simulink model "test_PCI6052E_20130416_3ch"  (Simulink 7.7)
settings: Solver=ode4  StartTime=0.0  StopTime=inf  RelTol=1e-3
PreLoadFcn:
  | % Here are parameters fixed
  | % during running the real-time programs.
  | %
  | winLen=256;
  | ana_hopSize=44;
  | syn_hopSize=90;
  | 
  | nFFT=1024;
  | SampRate=44100;
  | Ts=1/SampRate;
  | 
  | % % now encoded in RealSong_control
  | %cepst_nfft=2048;    % nfft size for cepstrum.
  | %
  | %up_pitch= 8000;%
  | %low_pitch=400;%
  | %
  | %quefrency = [0:cepst_nfft]'*nFFT/(SampRate*cepst_nfft); % quefrency in [sec].
  | %quefrency_index=find((1./quefrency<up_pitch & 1./quefrency > low_pitch)); % select quefrency in 400 to 8000 Hz range.
  | 
  | 
  | %frange=[400,8000];
  | %f=SampRate*((1:nFFT)-1)/nFFT;
  | %findex=find(f>=frange(1)&f<=frange(2));
  | %entropy_frange=[1000,8000];
  | %efindex=find(f>=entropy_frange(1)&f<=entropy_frange(2));
  | 
  | 
  | mingap=1;
  | minsyl =6;
values from neighbouring files (symbols this model uses):
  amp_thresh = str2double(get(handles.edit_amp_thresh,'String'))    [RealSong_control_013.m]
  efindex = find(f>=efrange(1)&f<=efrange(2))    [RealSong_control_013.m]
  findex = find(f>=pm.frange(1)&f<=pm.frange(2))    [RealSong_control_013.m]
  mainsyl = varargin{1}    [RealSong_control_013.m]
  quefrency_index = find((1./quefrency<up_pitch & 1./quefrency > low_pitch))    [RealSong_control_013.m]
  scaling_factor = presyl.template_scaling_factor    [RealSong_control_013.m]
undefined symbols (not defined in the file or in its folder): AO1_TTL_Freq, dfilt, init_stim_vector, maindetection_startcnt, maintarget_spectrum_filter, max_presyl_cancel_counter, presyl_cntmin, svmdata
libraries: simulink x13, dspsigops x4, xpcnilib x3, dsparch4 x2, dspxfrm3 x2
(part 2 of 2)

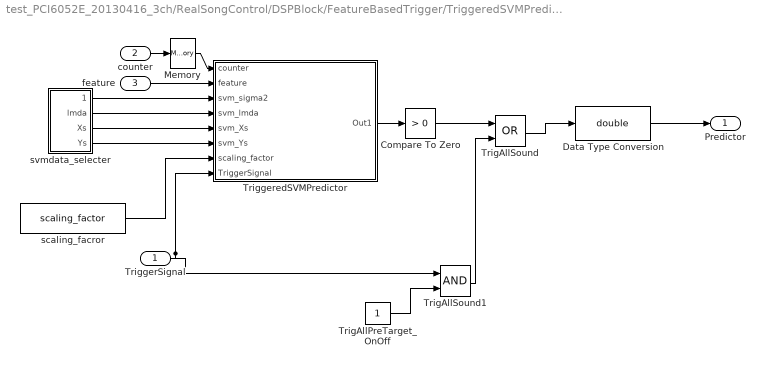
== system test_PCI6052E_20130416_3ch/RealSongControl/DSPBlock/FeatureBasedTrigger/TriggeredSVMPredictor ==
  TriggerSignal : Inport
  counter : Inport  Port=2
  feature : Inport  Port=3
  Compare To Zero : simulink/Logic and Bit Operations/Compare To Zero  SystemSampleTime=-1  relop=>  LogicOutDataTypeMode=uint8
  Data Type Conversion : DataTypeConversion  OutDataTypeStr=double
  Memory : Memory  InheritSampleTime=on
  TrigAllPreTarget_OnOff : Constant  VectorParams1D=off
  TrigAllSound : Logic  Operator=OR  AllPortsSameDT=off  OutDataTypeStr=boolean
  TrigAllSound1 : Logic  AllPortsSameDT=off  OutDataTypeStr=boolean
  TriggeredSVMPredictor : Subsystem  TreatAsAtomicUnit=on
  scaling_facror : Constant  Value=scaling_factor
  svmdata_selecter : Subsystem  mask{svmdata=svmdata}
      mask prompts: svmdata "svm data"
  Predictor : Outport
  wires:
  scaling_facror/1 -> TriggeredSVMPredictor/7(scaling_factor)
  svmdata_selecter/1(sigma2) -> TriggeredSVMPredictor/3(svm_sigma2)
  svmdata_selecter/2(lmda) -> TriggeredSVMPredictor/4(svm_lmda)
  svmdata_selecter/3(Xs) -> TriggeredSVMPredictor/5(svm_Xs)
  svmdata_selecter/4(Ys) -> TriggeredSVMPredictor/6(svm_Ys)
  counter/1 -> Memory/1
  feature/1 -> TriggeredSVMPredictor/2(feature)
  TriggeredSVMPredictor/1(Out1) -> Compare To Zero/1
  TriggerSignal/1 -> TriggeredSVMPredictor/8(TriggerSignal), TrigAllSound1/1
  Memory/1 -> TriggeredSVMPredictor/1(counter)
  Data Type Conversion/1 -> Predictor/1
  Compare To Zero/1 -> TrigAllSound/1
  TrigAllSound/1 -> Data Type Conversion/1
  TrigAllPreTarget_OnOff/1 -> TrigAllSound1/2
  TrigAllSound1/1 -> TrigAllSound/2

== system test_PCI6052E_20130416_3ch/RealSongControl/DSPBlock/FeatureBasedTrigger/amplitude triggered  Iterative_mean_var ==
  note: 1: entropy
      | 2: FM
      | 3: frequency
      | 4: pitch
      | 5: pitchgoodness
  amp : Inport
  features : Inport  Port=2
  amp_thresh : Inport  Port=3
  AboveAmplitudeDetectionAndCounter1 : Subsystem  mask{mingap=mingap, minsyl=minsyl}
      mask prompts: mingap "Gap shorter than this is neglected"; minsyl "On state must be longer than this"
  AboveSyllableCounter : Subsystem
  Iterative_mean_var : Stateflow chart  TreatAsAtomicUnit=on
  on_signal : Outport
  syl_duration : Outport  Port=2
  meanvar : Outport  Port=3
  wires:
  Iterative_mean_var/1(out) -> meanvar/1
  features/1 -> Iterative_mean_var/1(x)
  amp/1 -> AboveAmplitudeDetectionAndCounter1/1(Input)
  amp_thresh/1 -> AboveAmplitudeDetectionAndCounter1/2(threshold)
  AboveAmplitudeDetectionAndCounter1/1(SignalOn) -> Iterative_mean_var/2(on_signal), on_signal/1, AboveSyllableCounter/1(LogicalInput)
  AboveSyllableCounter/1(count) -> syl_duration/1

== system test_PCI6052E_20130416_3ch/RealSongControl/DSPBlock/SoundOnOffCounter/SoundOffCounter ==
  LogicalInput : Inport
  Counter : Subsystem  TreatAsAtomicUnit=on
  Data Type Conversion1 : DataTypeConversion  OutDataTypeStr=double  RndMeth=Zero
  count : Outport
  wires:
  Data Type Conversion1/1 -> Counter/1(In1)
  LogicalInput/1 -> Data Type Conversion1/1, Counter/Enable
  Counter/1(Out1) -> count/1

== system test_PCI6052E_20130416_3ch/RealSongControl/DSPBlock/SoundOnOffCounter/SoundOnCounter ==
  LogicalInput : Inport
  Counter : Subsystem  TreatAsAtomicUnit=on
  Data Type Conversion1 : DataTypeConversion  OutDataTypeStr=double  RndMeth=Zero
  count : Outport
  wires:
  Data Type Conversion1/1 -> Counter/1(In1)
  LogicalInput/1 -> Data Type Conversion1/1, Counter/Enable
  Counter/1(Out1) -> count/1

== system test_PCI6052E_20130416_3ch/RealSongControl/DSPBlock/BoutCounter/BoutDurCounter/CorrectDelayedPulseGenerator ForSyllableOn ==
  trig : Inport
  DSP Constant2 : Constant  Value=maindetection_startcnt  VectorParams1D=off
  DSP Constant3 : Constant  Value=width  VectorParams1D=off
  Delayed TTL generator : Stateflow chart  TreatAsAtomicUnit=on
  TTL : Outport
  wires:
  DSP Constant2/1 -> Delayed TTL generator/2(delays)
  DSP Constant3/1 -> Delayed TTL generator/3(width)
  trig/1 -> Delayed TTL generator/1(trig)
  Delayed TTL generator/1(out) -> TTL/1

== system test_PCI6052E_20130416_3ch/RealSongControl/DSPBlock/BoutCounter/BoutDurCounter/PreSoundOnCounter ==
  LogicalInput : Inport
  Counter : Subsystem  TreatAsAtomicUnit=on
  Data Type Conversion1 : DataTypeConversion  OutDataTypeStr=double  RndMeth=Zero
  count : Outport
  wires:
  Data Type Conversion1/1 -> Counter/1(In1)
  LogicalInput/1 -> Data Type Conversion1/1, Counter/Enable
  Counter/1(Out1) -> count/1

== system test_PCI6052E_20130416_3ch/RealSongControl/DSPBlock/BoutCounter/BoutDurCounter/SoundOnCounter ==
  LogicalInput : Inport
  Counter : Subsystem  TreatAsAtomicUnit=on
  Data Type Conversion1 : DataTypeConversion  OutDataTypeStr=double  RndMeth=Zero
  count : Outport
  wires:
  Data Type Conversion1/1 -> Counter/1(In1)
  LogicalInput/1 -> Data Type Conversion1/1, Counter/Enable
  Counter/1(Out1) -> count/1

== system test_PCI6052E_20130416_3ch/RealSongControl/DSPBlock/FeatureBasedTrigger/MainDetectCounter/Counter ==
  In1 : Inport
  Enable : EnablePort  StatesWhenEnabling=reset
  Memory1 : Memory  InheritSampleTime=on
  Sum1 : Sum  Inputs=|++  SaturateOnIntegerOverflow=on
  Out1 : Outport  OutputWhenDisabled=reset  InitialOutput=0
  wires:
  In1/1 -> Sum1/1
  Sum1/1 -> Out1/1, Memory1/1
  Memory1/1 -> Sum1/2

== system test_PCI6052E_20130416_3ch/RealSongControl/DSPBlock/FeatureBasedTrigger/PreSyllableDetectionAtEndOfSyllable/CancelCounter ==
  LogicalInput : Inport
  Counter : Subsystem  TreatAsAtomicUnit=on
  Data Type Conversion1 : DataTypeConversion  OutDataTypeStr=double  RndMeth=Zero
  count : Outport
  wires:
  Data Type Conversion1/1 -> Counter/1(In1)
  LogicalInput/1 -> Data Type Conversion1/1, Counter/Enable
  Counter/1(Out1) -> count/1

== system test_PCI6052E_20130416_3ch/RealSongControl/DSPBlock/FeatureBasedTrigger/PreSyllableDetectionAtEndOfSyllable/EnabledKeepMaxCounter ==
  enable : Inport
  binarysignal : Inport  Port=2
  EnabledMaxCounter : Subsystem  TreatAsAtomicUnit=on
  SyllableCounter : Subsystem
  MaxCount : Outport
  wires:
  SyllableCounter/1(count) -> EnabledMaxCounter/1(In1)
  enable/1 -> EnabledMaxCounter/Enable
  EnabledMaxCounter/1(Out1) -> MaxCount/1
  binarysignal/1 -> SyllableCounter/1(LogicalInput)

== system test_PCI6052E_20130416_3ch/RealSongControl/DSPBlock/FeatureBasedTrigger/RndCatchMainGateWindow/CorrectDelayedPulseGenerator ==
  trig : Inport
  delay : Inport  Port=2
  width : Inport  Port=3
  Delayed TTL generator : Stateflow chart  TreatAsAtomicUnit=on
  TTL : Outport
  wires:
  delay/1 -> Delayed TTL generator/2(delays)
  width/1 -> Delayed TTL generator/3(width)
  trig/1 -> Delayed TTL generator/1(trig)
  Delayed TTL generator/1(out) -> TTL/1

== system test_PCI6052E_20130416_3ch/RealSongControl/DSPBlock/FeatureBasedTrigger/RndCatchMainGateWindow/CorrectDelayedPulseGenerator1 ==
  trig : Inport
  delay : Inport  Port=2
  width : Inport  Port=3
  Delayed TTL generator : Stateflow chart  TreatAsAtomicUnit=on
  TTL : Outport
  wires:
  delay/1 -> Delayed TTL generator/2(delays)
  width/1 -> Delayed TTL generator/3(width)
  trig/1 -> Delayed TTL generator/1(trig)
  Delayed TTL generator/1(out) -> TTL/1

== system test_PCI6052E_20130416_3ch/RealSongControl/DSPBlock/FeatureBasedTrigger/RndCatchMainGateWindow/EnabledCatchSignalBox ==
  In1 : Inport
  Enable : EnablePort
  CatchLine : Logic  Operator=NOT  AllPortsSameDT=off  OutDataTypeStr=boolean
  CatchRatioConstant : Constant  Value=0
  PreSyllableDetection : Logic  AllPortsSameDT=off  OutDataTypeStr=boolean
  Relational Operator : RelationalOperator  Operator=<=  OutDataTypeStr=boolean
  Uniform Random Number : UniformRandomNumber  Minimum=0
  Hit : Outport  OutputWhenDisabled=reset  InitialOutput=0
  Catch : Outport  Port=2  OutputWhenDisabled=reset  InitialOutput=0
  wires:
  CatchRatioConstant/1 -> Relational Operator/1
  Uniform Random Number/1 -> Relational Operator/2
  PreSyllableDetection/1 -> Hit/1, CatchLine/1
  In1/1 -> PreSyllableDetection/1
  Relational Operator/1 -> PreSyllableDetection/2
  CatchLine/1 -> Catch/1

== system test_PCI6052E_20130416_3ch/RealSongControl/DSPBlock/FeatureBasedTrigger/TriggeredSVMPredictor/TriggeredSVMPredictor ==
  counter : Inport
  feature : Inport  Port=2
  svm_sigma2 : Inport  Port=3
  svm_lmda : Inport  Port=4
  svm_Xs : Inport  Port=5
  svm_Ys : Inport  Port=6
  scaling_factor : Inport  Port=7
  TriggerSignal : Inport  Port=8
  svm_predict : Stateflow chart  TreatAsAtomicUnit=on
  Out1 : Outport
  wires:
  counter/1 -> svm_predict/1(counter)
  svm_predict/1(predictor) -> Out1/1
  feature/1 -> svm_predict/2(feature)
  svm_sigma2/1 -> svm_predict/3(svm_sigma2)
  svm_lmda/1 -> svm_predict/4(svm_lmda)
  svm_Xs/1 -> svm_predict/5(svm_Xs)
  svm_Ys/1 -> svm_predict/6(svm_Ys)
  scaling_factor/1 -> svm_predict/7(scaling_factor)
  TriggerSignal/1 -> svm_predict/8(trig)

== system test_PCI6052E_20130416_3ch/RealSongControl/DSPBlock/FeatureBasedTrigger/TriggeredSVMPredictor/svmdata_selecter ==
  svmdata : Constant  Value=svmdata.lmda
  svmdata1 : Constant  Value=svmdata.sigma2
  svmdata2 : Constant  Value=svmdata.Ys
  svmdata3 : Constant  Value=svmdata.Xs
  sigma2 : Outport
  lmda : Outport  Port=2
  Xs : Outport  Port=3
  Ys : Outport  Port=4
  wires:
  svmdata1/1 -> sigma2/1
  svmdata/1 -> lmda/1
  svmdata3/1 -> Xs/1
  svmdata2/1 -> Ys/1

== system test_PCI6052E_20130416_3ch/RealSongControl/DSPBlock/FeatureBasedTrigger/amplitude triggered  Iterative_mean_var/AboveAmplitudeDetectionAndCounter1 ==
  Input : Inport
  threshold : Inport  Port=2
  CorrectDelayedPulseGenerator ForSyllableOn : Subsystem  mask{maindetection_startcnt=0, width=mingap}
      mask prompts: maindetection_startcnt "Delay (count)"; width "Width of TTL (count)"
  DSP Constant2 : Constant  Value=minsyl  VectorParams1D=off
  PreSoundOnCounter : Subsystem
  Relational Operator : RelationalOperator  Operator=>  OutDataTypeStr=boolean
  Relational Operator1 : RelationalOperator  Operator=>  OutDataTypeStr=boolean
  SoundOnCounter : Subsystem
  SignalOn : Outport
  SignalOnCnt : Outport  Port=2
  wires:
  Relational Operator/1 -> CorrectDelayedPulseGenerator ForSyllableOn/1(trig)
  Input/1 -> Relational Operator/1
  threshold/1 -> Relational Operator/2
  CorrectDelayedPulseGenerator ForSyllableOn/1(TTL) -> PreSoundOnCounter/1(LogicalInput)
  PreSoundOnCounter/1(count) -> Relational Operator1/1
  Relational Operator1/1 -> SignalOn/1, SoundOnCounter/1(LogicalInput)
  DSP Constant2/1 -> Relational Operator1/2
  SoundOnCounter/1(count) -> SignalOnCnt/1

== system test_PCI6052E_20130416_3ch/RealSongControl/DSPBlock/FeatureBasedTrigger/amplitude triggered  Iterative_mean_var/AboveSyllableCounter ==
  LogicalInput : Inport
  Counter : Subsystem  TreatAsAtomicUnit=on
  Data Type Conversion1 : DataTypeConversion  OutDataTypeStr=double  RndMeth=Zero
  count : Outport
  wires:
  Data Type Conversion1/1 -> Counter/1(In1)
  LogicalInput/1 -> Data Type Conversion1/1, Counter/Enable
  Counter/1(Out1) -> count/1

== system test_PCI6052E_20130416_3ch/RealSongControl/DSPBlock/SoundOnOffCounter/SoundOffCounter/Counter ==
  In1 : Inport
  Enable : EnablePort  StatesWhenEnabling=reset
  Memory1 : Memory  InheritSampleTime=on
  Sum1 : Sum  Inputs=|++  SaturateOnIntegerOverflow=on
  Out1 : Outport  OutputWhenDisabled=reset  InitialOutput=0
  wires:
  In1/1 -> Sum1/1
  Sum1/1 -> Out1/1, Memory1/1
  Memory1/1 -> Sum1/2

== system test_PCI6052E_20130416_3ch/RealSongControl/DSPBlock/SoundOnOffCounter/SoundOnCounter/Counter ==
  In1 : Inport
  Enable : EnablePort  StatesWhenEnabling=reset
  Memory1 : Memory  InheritSampleTime=on
  Sum1 : Sum  Inputs=|++  SaturateOnIntegerOverflow=on
  Out1 : Outport  OutputWhenDisabled=reset  InitialOutput=0
  wires:
  In1/1 -> Sum1/1
  Sum1/1 -> Out1/1, Memory1/1
  Memory1/1 -> Sum1/2

== system test_PCI6052E_20130416_3ch/RealSongControl/DSPBlock/BoutCounter/BoutDurCounter/PreSoundOnCounter/Counter ==
  In1 : Inport
  Enable : EnablePort  StatesWhenEnabling=reset
  Memory1 : Memory  InheritSampleTime=on
  Sum1 : Sum  Inputs=|++  SaturateOnIntegerOverflow=on
  Out1 : Outport  OutputWhenDisabled=reset  InitialOutput=0
  wires:
  In1/1 -> Sum1/1
  Sum1/1 -> Out1/1, Memory1/1
  Memory1/1 -> Sum1/2

== system test_PCI6052E_20130416_3ch/RealSongControl/DSPBlock/BoutCounter/BoutDurCounter/SoundOnCounter/Counter ==
  In1 : Inport
  Enable : EnablePort  StatesWhenEnabling=reset
  Memory1 : Memory  InheritSampleTime=on
  Sum1 : Sum  Inputs=|++  SaturateOnIntegerOverflow=on
  Out1 : Outport  OutputWhenDisabled=reset  InitialOutput=0
  wires:
  In1/1 -> Sum1/1
  Sum1/1 -> Out1/1, Memory1/1
  Memory1/1 -> Sum1/2

== system test_PCI6052E_20130416_3ch/RealSongControl/DSPBlock/FeatureBasedTrigger/PreSyllableDetectionAtEndOfSyllable/CancelCounter/Counter ==
  In1 : Inport
  Enable : EnablePort  StatesWhenEnabling=reset
  Memory1 : Memory  InheritSampleTime=on
  Sum1 : Sum  Inputs=|++  SaturateOnIntegerOverflow=on
  Out1 : Outport  OutputWhenDisabled=reset  InitialOutput=0
  wires:
  In1/1 -> Sum1/1
  Sum1/1 -> Out1/1, Memory1/1
  Memory1/1 -> Sum1/2

== system test_PCI6052E_20130416_3ch/RealSongControl/DSPBlock/FeatureBasedTrigger/PreSyllableDetectionAtEndOfSyllable/EnabledKeepMaxCounter/EnabledMaxCounter ==
  In1 : Inport
  Enable : EnablePort  StatesWhenEnabling=reset
  Memory : Memory  InheritSampleTime=on
  MinMax : MinMax  Function=max  Inputs=2
  Out1 : Outport  OutputWhenDisabled=reset  InitialOutput=0
  wires:
  In1/1 -> MinMax/1
  MinMax/1 -> Out1/1, Memory/1
  Memory/1 -> MinMax/2

== system test_PCI6052E_20130416_3ch/RealSongControl/DSPBlock/FeatureBasedTrigger/PreSyllableDetectionAtEndOfSyllable/EnabledKeepMaxCounter/SyllableCounter ==
  LogicalInput : Inport
  Counter : Subsystem  TreatAsAtomicUnit=on
  Data Type Conversion1 : DataTypeConversion  OutDataTypeStr=double  RndMeth=Zero
  count : Outport
  wires:
  Data Type Conversion1/1 -> Counter/1(In1)
  LogicalInput/1 -> Data Type Conversion1/1, Counter/Enable
  Counter/1(Out1) -> count/1

== system test_PCI6052E_20130416_3ch/RealSongControl/DSPBlock/FeatureBasedTrigger/amplitude triggered  Iterative_mean_var/AboveAmplitudeDetectionAndCounter1/CorrectDelayedPulseGenerator ForSyllableOn ==
  trig : Inport
  DSP Constant2 : Constant  Value=maindetection_startcnt  VectorParams1D=off
  DSP Constant3 : Constant  Value=width  VectorParams1D=off
  Delayed TTL generator : Stateflow chart  TreatAsAtomicUnit=on
  TTL : Outport
  wires:
  DSP Constant2/1 -> Delayed TTL generator/2(delays)
  DSP Constant3/1 -> Delayed TTL generator/3(width)
  trig/1 -> Delayed TTL generator/1(trig)
  Delayed TTL generator/1(out) -> TTL/1

== system test_PCI6052E_20130416_3ch/RealSongControl/DSPBlock/FeatureBasedTrigger/amplitude triggered  Iterative_mean_var/AboveAmplitudeDetectionAndCounter1/PreSoundOnCounter ==
  LogicalInput : Inport
  Counter : Subsystem  TreatAsAtomicUnit=on
  Data Type Conversion1 : DataTypeConversion  OutDataTypeStr=double  RndMeth=Zero
  count : Outport
  wires:
  Data Type Conversion1/1 -> Counter/1(In1)
  LogicalInput/1 -> Data Type Conversion1/1, Counter/Enable
  Counter/1(Out1) -> count/1

== system test_PCI6052E_20130416_3ch/RealSongControl/DSPBlock/FeatureBasedTrigger/amplitude triggered  Iterative_mean_var/AboveAmplitudeDetectionAndCounter1/SoundOnCounter ==
  LogicalInput : Inport
  Counter : Subsystem  TreatAsAtomicUnit=on
  Data Type Conversion1 : DataTypeConversion  OutDataTypeStr=double  RndMeth=Zero
  count : Outport
  wires:
  Data Type Conversion1/1 -> Counter/1(In1)
  LogicalInput/1 -> Data Type Conversion1/1, Counter/Enable
  Counter/1(Out1) -> count/1

== system test_PCI6052E_20130416_3ch/RealSongControl/DSPBlock/FeatureBasedTrigger/amplitude triggered  Iterative_mean_var/AboveSyllableCounter/Counter ==
  In1 : Inport
  Enable : EnablePort  StatesWhenEnabling=reset
  Memory1 : Memory  InheritSampleTime=on
  Sum1 : Sum  Inputs=|++  SaturateOnIntegerOverflow=on
  Out1 : Outport  OutputWhenDisabled=reset  InitialOutput=0
  wires:
  In1/1 -> Sum1/1
  Sum1/1 -> Out1/1, Memory1/1
  Memory1/1 -> Sum1/2

== system test_PCI6052E_20130416_3ch/RealSongControl/DSPBlock/FeatureBasedTrigger/PreSyllableDetectionAtEndOfSyllable/EnabledKeepMaxCounter/SyllableCounter/Counter ==
  In1 : Inport
  Enable : EnablePort  StatesWhenEnabling=reset
  Memory1 : Memory  InheritSampleTime=on
  Sum1 : Sum  Inputs=|++  SaturateOnIntegerOverflow=on
  Out1 : Outport  OutputWhenDisabled=reset  InitialOutput=0
  wires:
  In1/1 -> Sum1/1
  Sum1/1 -> Out1/1, Memory1/1
  Memory1/1 -> Sum1/2

== system test_PCI6052E_20130416_3ch/RealSongControl/DSPBlock/FeatureBasedTrigger/amplitude triggered  Iterative_mean_var/AboveAmplitudeDetectionAndCounter1/PreSoundOnCounter/Counter ==
  In1 : Inport
  Enable : EnablePort  StatesWhenEnabling=reset
  Memory1 : Memory  InheritSampleTime=on
  Sum1 : Sum  Inputs=|++  SaturateOnIntegerOverflow=on
  Out1 : Outport  OutputWhenDisabled=reset  InitialOutput=0
  wires:
  In1/1 -> Sum1/1
  Sum1/1 -> Out1/1, Memory1/1
  Memory1/1 -> Sum1/2

== system test_PCI6052E_20130416_3ch/RealSongControl/DSPBlock/FeatureBasedTrigger/amplitude triggered  Iterative_mean_var/AboveAmplitudeDetectionAndCounter1/SoundOnCounter/Counter ==
  In1 : Inport
  Enable : EnablePort  StatesWhenEnabling=reset
  Memory1 : Memory  InheritSampleTime=on
  Sum1 : Sum  Inputs=|++  SaturateOnIntegerOverflow=on
  Out1 : Outport  OutputWhenDisabled=reset  InitialOutput=0
  wires:
  In1/1 -> Sum1/1
  Sum1/1 -> Out1/1, Memory1/1
  Memory1/1 -> Sum1/2

== matlab function RealSongControl/triggered_signal_source_Song/Delayed_Triggered_Counter ==
  data: trig input double; delay input double; start_cnt input double; end_cnt input double; out output double; max_cnt input double; ref input double
function out = trig_counter(trig,delay,start_cnt,end_cnt,max_cnt,ref)
%#eml
% % Delayed Triggered Counter:
% 1) When not triggered, output value is max_cnt.
% 2 )Once triggered, output remains max_cnt during delay count period, 
% 3) then it starts to count from Start_Cnt to End_Cnt, 
% 4) After End_Cnt, it jumps to Max_Cnt.
% 
% This code is to select song stimli uploaded in the form of 
% a vector. For example, if OutValues_and_zero contains
% 3 song stimli, indexing from 1:1000,1001:2000, and 2001:4000,
% and if you want to drive second song, you can set Start_Cnt to 1001, End_Cnt to 2000.
% max_cnt needs to be length(OutValues_and_zero)+1 to make sure
% the analog output goes back to zero. 
% % It will not be triggered again until counter reaches to max_cnt. 

persistent delay_cnt; % counter 
persistent cnt; % counter 
persistent ref_cnt; % refractoriness counter 


if isempty(cnt)
    cnt         = max_cnt;
    ref_cnt     = inf;
    delay_cnt   = inf;
end

if (trig>0) && (cnt>=max_cnt) && (ref_cnt>ref)
    cnt=start_cnt;
    ref_cnt=0;
    delay_cnt=0;
end

delay_cnt = delay_cnt+1;

if delay_cnt>=delay
   delay_cnt=delay +1; % Fix the delay count.
   cnt=cnt+1; 
   ref_cnt=ref_cnt+1;
end

if cnt>=end_cnt
    cnt=max_cnt;
end


if ref_cnt>ref
    ref_cnt=ref+1; % Fix the refractoriness count.
end

out=cnt;

== matlab function RealSongControl/DSPBlock/Multitaper_Feature/multitaper_feature_RTSAC ==
  data: J1 input double; J2 input double; Ts input double; findex input double; m_amplitude output double; m_Entropy output double; m_FM output double; m_frequency output double; m_Pitch output double; m_PitchGoodness output double; m_PrecisePitch output double; efindex input double; m_time_deriv_max output double; m_freq_deriv_max output double; quefrency_select input double; m_powSpec_findex output double
function [  m_amplitude,...
            m_Entropy,...
            m_FM,...
            m_frequency,...
            m_Pitch,...
            m_PitchGoodness,...
            m_PrecisePitch,...
            m_time_deriv_max,...
            m_freq_deriv_max,...
            m_powSpec_findex] = multitaper_feature_RTSAC(J1,J2,Ts,...
            findex,efindex,quefrency_select)
% J1: taper1 windowed FFT signal, column vector.
% J2: taper2 windowed FFT signal, column vector.
% Ts: sample time 
% frange: frequency range to take into consider
% [  m_spec_deriv,...
%             m_amplitude,...
%             m_Entropy,...
%             m_FM,...
%             m_AM,...
%             m_frequency,...
%             m_Pitch,...
%             m_PitchGoodness] = multitaper_feature_RTSAC(J1,J2,Ts,nFFT)
%  This is a copy of multitaper_feature_RTSAC.m
% by KH 20120104
% frange=[400,8000];

% nfft size for frequency calculation. When you change this,
% please also change the value in RealSong_control

nFFT=1024;
fs=1/Ts;
f=fs*((1:nFFT)-1)/nFFT;

% nfft size for cepstrum. When you change this,
% please also change the value in RealSong_control
cepst_nfft=2048;   


% In this code, findex, efindex, quefrency_index are given.

% % frange=[400,10000];
% findex=find(f>=frange(1)&f<=frange(2));
% entropy_frange=[1000,8000];
% efindex=find(f>=entropy_frange(1)&f<=entropy_frange(2));

%==============Power spectrum=============

m_powSpec=real(J1.*conj(J1)+(J2.*conj(J2)));


m_time_deriv=-real(J1.*conj(J2));
% m_time_deriv=-real(J1).*real(J2)-imag(J1).*imag(J2);
m_freq_deriv=-real(conj(J1*1i).*J2);
% m_freq_deriv=+imag(J1).*real(J2)-real(J1).*imag(J2);

m_time_deriv_max=max(m_time_deriv(findex).^2,[],1);
m_freq_deriv_max=max(m_freq_deriv(findex).^2,[],1);

%===

m_amplitude=real(sum(m_powSpec(findex)));

log_power=m_time_deriv(findex).^2+m_freq_deriv(findex).^2;
m_SumLog=sum(log(m_powSpec(efindex)));
m_LogSum=mean(m_powSpec(efindex));

m_frequency=(f(findex)*log_power)/(sum(log_power)+eps);
% gc_base=sum(log_power);
% m_AM=sum(m_time_deriv(findex));


% m_frequency=m_frequency./max(gc_base,1)*fs/pad;
% m_frequency=Nyq*m_frequency./(gc_base+eps)/length(findex);
% m_AM=m_AM./(m_amplitude+eps);
m_amplitude=log10(m_amplitude+1)*10; %units in Db


%===========Wiener entropy==================
if m_LogSum==0
    m_LogSum=0;
    m_Entropy=0;
else
    m_LogSum=log(m_LogSum); %divide by the number of frequencies
    m_Entropy=(m_SumLog/length(efindex))-m_LogSum;
end




%============FM===================

m_FM=real(atan(m_time_deriv_max/(m_freq_deriv_max+eps)));
%m_FM(find(m_freq_deriv_max==0))=0;

%%%%%%%%%%%%%%%%%%%%%%%%

%==========Directional Spectral derivatives=================

% 
cFM=cos(m_FM);
sFM=sin(m_FM);

%==The image==
m_spec_deriv=sFM*m_time_deriv(findex)+cFM*m_freq_deriv(findex);
% Cepstrum=(fft(m_spec_deriv./(m_powSpec(3:255)+eps),512,2))*( 1/2);
% % Cepstrum=fft(abs(m_spec_deriv),512,2);
% m_spec_deriv=m_powSpec(findex);

pitch_HoP=1800;%hz
gdn_HoP=10;
up_wiener=-1;

Cepstrum=fft(m_spec_deriv(3:end)./(m_powSpec(findex(3:end))+eps),cepst_nfft)*( 1/2);

x=abs(Cepstrum(quefrency_select)).^2;
bias=3;
[m_PitchGoodness,m]=max(x(bias:end));
m=m+bias-1;
m_Pitch= 1 / (m*nFFT/(fs*cepst_nfft)); % Hz.


df=1;
if m==1 
    parabolic_estimate_m = 1;
elseif m==length(x)
    parabolic_estimate_m = 1;
else   
    dy1 = x(m-1)-x(m);
    dy2 = x(m)-x(m+1);
    
    a = -(dy1-dy2)/(2*df^2);
    b = dy1/df - 2 * a * (m-0.5);
    parabolic_estimate_m = -b/(2*a);
end
% fprintf('Cubic estimated of auto-correlation peak is %3.5gsec (freq=%3.5g)\n',...
%     cubic_estime_t,1/cubic_estime_t);
m_PrecisePitch= 1 / (parabolic_estimate_m*nFFT/(fs*cepst_nfft));

% if pitch is too high or goodness of pitch is too low, and entropy is too
% high (noisy), just use frequency as pitch value.
if ((m_Pitch>pitch_HoP) || (m_PitchGoodness<gdn_HoP)) &&( m_Entropy>up_wiener)
    m_Pitch=m_frequency;
end

m_FM=m_FM*180/pi;

m_powSpec_findex=m_powSpec(findex);
m_powSpec_findex=m_powSpec_findex/sum(m_powSpec_findex);

== matlab function RealSongControl/DSPBlock/FeatureBasedTrigger/RndCatchMainGateWindow/CorrectDelayedPulseGenerator/Delayed TTL generator ==
  data: trig input double; out output double; delays input double; width input double
function out = fcn(trig,delays,width)
% return delayed broader TTL pulse.
% Trigger always reset the delay counter, therefore, 
% when two trigger occurs, first one can be just forgotten. 
% by KH.

persistent cnt_for_delay; % counter for delays
persistent width_cnt;


if isempty(cnt_for_delay)
    cnt_for_delay=-inf(size(trig));
    width_cnt=zeros(size(trig));
end

cnt_for_delay=cnt_for_delay-1;
trigind=(trig>0);

width_cnt(cnt_for_delay==0)=width; % set width counter.
cnt_for_delay(trigind)=delays(trigind)+1; % plus one, so that delays=0 can trigger next time.

width_cnt=width_cnt-1;    
out=(width_cnt>0);

== matlab function RealSongControl/DSPBlock/FeatureBasedTrigger/amplitude triggered Iterative_mean_var/Iterative_mean_var ==
  data: x input double; out output double; on_signal input double
function out =triggered_iterative_mean_var(x,on_signal)
%#eml
% estimate mean and variance from the continuously flowing-in data,
% by using the iterative relationship.
%
% %ex)
% --- init---
% iterative_mean_var([],-1)
% --- estimate ---
% out=iterative_mean_var(x,1);
% where x is Nx1 vector;
% out is the 2Nx1 vector with
% first N are mean of x, next N are var of x.
%
% if no data available, put zero vector with the same size,
% or iterative_mean_var([],'reset').
%
% 'init':  initiallize and construct internal variables
% 'reset': just reset internal variables without constructing it
%
%
% --- iterative method to calculate mean and variance ---
% E(x_n)  =(N-1)/N*E(x_{n-1})+1/N*x_n;
% E(x_n^2)=(N-1)/N*E(x_{n-1}^2)+1/N*x_n^2;
% V(x_n)  =E(x_n^2) - E(x_n)^2;
%
%
% ex)
% x=zeros(4,1);
% iterative_mean_var(x,'init');
% out=zeros(8,100);
% for ii=1:100
% if mod(ii,20)==0, x=0; else x=[-70,0.5,10,50]'+randn(4,1);end
% out(:,ii)=iterative_mean_var(x);
% end
% plot(out')
% by KH 20101027

persistent cnt tmp tmp2 tmpout

if isempty(cnt)
    tmp=zeros(length(x),1);
    tmp2=zeros(length(x),1);
    tmpout=zeros(2*length(x),1);
    cnt=0;
end


if on_signal>0 % Start mean and var calculation
    
    if all(x==0)
        cnt=0;
        tmp=zeros(length(tmp),1);
        tmp2=zeros(length(tmp2),1);
        tmpout=zeros(2*length(tmp),1);
        
    else
        cnt=cnt+1;
        
        tmp=(cnt-1)/cnt*tmp     +x/cnt;
        tmp2=(cnt-1)/cnt*tmp2   +(x.^2)/cnt;
       
        tmpout(1:length(x))= tmp;
        tmpout((length(x)+1):end)=tmp2-tmp.^2;
        
    end
    
else
    
    tmp=zeros(length(x),1);
    tmp2=zeros(length(x),1);
    tmpout=zeros(2*length(x),1);
    cnt=0;
end

out=tmpout;

== matlab function RealSongControl/DSPBlock/FeatureBasedTrigger/TriggeredSVMPredictor/TriggeredSVMPredictor/svm_predict ==
  data: counter input double; feature input double; svm_sigma2 input double; svm_lmda input double; svm_Xs input double; svm_Ys input double; predictor output double; scaling_factor input double; trig input double
function predictor= svm_predict(counter,...
    feature,...
    svm_sigma2,...
    svm_lmda,...
    svm_Xs,...
    svm_Ys,...
    scaling_factor,...
    trig)
%#eml

predictor=double(0);

if trig>0
    
sv.sigma2=svm_sigma2;
sv.lmda=svm_lmda;
sv.Xs  =svm_Xs;
sv.Ys  =svm_Ys;


tmp_features=[counter;feature];
x=tmp_features./scaling_factor;
% [g_predict,b] = my_predictsvm(sv, x);
% predictor=g_predict-b;

predictor=my_predictsvm_neglect_bias(sv, x);
end

%-----------------------------------------------------------------------%
function [g,b] = my_predictsvm(sv,X)
% [maxlmda,ind]=max(sv.lmda);



nsample=size(sv.Xs,2);
dot_xs = sum(sv.Xs.*sv.Xs,1);
XiXj    = sv.Xs'*sv.Xs;
unit_vec = ones(1,nsample);

K=zeros(nsample);
for ii=1:nsample
    %     K(ii,:)= exp(sigma2*(2*XiXj(ii,:)-dot_x-dot_x(ii)*unit_vec)).*;
    K(ii,:)= exp(sv.sigma2*...
        (2*XiXj(ii,:)-dot_xs-dot_xs(ii)*unit_vec));
end

b=mean(sv.Ys(:)-K*(sv.lmda.*sv.Ys));
    
    

  dot_X = sum(X.*X,1);
  xxs =  X'*sv.Xs;
  
  K =  exp(sv.sigma2 *...
        (2 * xxs - dot_xs(ones(size(X,2),1),:) - repmat(dot_X(:),1,nsample)))...
        *(sv.lmda.*sv.Ys);
  
% get prediction   
g = b + K;



%---------------------------------------------------%
%--- modified code, assuming X is a column vector ---%
function [K] = my_predictsvm_neglect_bias(sv,X)
% [maxlmda,ind]=max(sv.lmda);
persistent dot_xs; 
persistent XiXj;

if isempty(dot_xs)
    % nsample=size(sv.Xs,2);
    dot_xs = sum(sv.Xs.*sv.Xs,1);
    XiXj    = sv.Xs'*sv.Xs;
    % unit_vec = ones(1,nsample);
end


% K=zeros(nsample);
% for ii=1:nsample
%     %     K(ii,:)= exp(sigma2*(2*XiXj(ii,:)-dot_x-dot_x(ii)*unit_vec)).*;
%     K(ii,:)= exp(sv.sigma2*...
%         (2*XiXj(ii,:)-dot_xs-dot_xs(ii)*unit_vec));
% end

% b=mean(sv.Ys(:)-K*(sv.lmda.*sv.Ys));
    
    

  dot_X = X'*X;
  xxs =  X'*sv.Xs;
  
  K =  exp(sv.sigma2 * (2 * xxs - dot_xs - dot_X)) *(sv.lmda.*sv.Ys);
  
% get prediction   
% g = b + K;

== matlab function RealSongControl/DSPBlock/FeatureBasedTrigger/amplitude triggered Iterative_mean_var/AboveAmplitudeDetectionAndCounter1/CorrectDelayedPulseGenerator ForSyllableOn/Delayed TTL generator ==
  data: trig input double; out output double; delays input double; width input double
function out = fcn(trig,delays,width)
% return delayed broader TTL pulse, 
% 
% 
persistent cnt_for_delay; % counter for delays
persistent width_cnt;


if isempty(cnt_for_delay)
    cnt_for_delay=-inf(size(trig));
    width_cnt=zeros(size(trig));
end

cnt_for_delay=cnt_for_delay-1;
trigind=(trig>0);

width_cnt(cnt_for_delay==0)=width; % set width counter.
cnt_for_delay(trigind)=delays(trigind)+1; % plus one, so that delays=0 can trigger next time.

width_cnt=width_cnt-1;    
out=(width_cnt>=0);

== matlab function OscilloAntidromic/CorrectDelayedPulseGenerator/Delayed TTL generator ==
  data: trig input double; out output double; delays input double; width input double
function out = fcn(trig,delays,width)
% return delayed broader TTL pulse, 
% 
% 
persistent cnt_for_delay; % counter for delays
persistent width_cnt;


if isempty(cnt_for_delay)
    cnt_for_delay=-inf(size(trig));
    width_cnt=zeros(size(trig));
end

cnt_for_delay=cnt_for_delay-1;
trigind=(trig>0);

width_cnt(cnt_for_delay==0)=width; % set width counter.
cnt_for_delay(trigind)=delays(trigind)+1; % plus one, so that delays=0 can trigger next time.

width_cnt=width_cnt-1;    
out=(width_cnt>0);

== matlab function RealSongControl/DSPBlock/BoutCounter/BoutDurCounter/CorrectDelayedPulseGenerator ForSyllableOn/Delayed TTL generator ==
  data: trig input double; out output double; delays input double; width input double
function out = fcn(trig,delays,width)
% return delayed broader TTL pulse, 
% 
% 
persistent cnt_for_delay; % counter for delays
persistent width_cnt;


if isempty(cnt_for_delay)
    cnt_for_delay=-inf(size(trig));
    width_cnt=zeros(size(trig));
end

cnt_for_delay=cnt_for_delay-1;
trigind=(trig>0);

width_cnt(cnt_for_delay==0)=width; % set width counter.
cnt_for_delay(trigind)=delays(trigind)+1; % plus one, so that delays=0 can trigger next time.

width_cnt=width_cnt-1;    
out=(width_cnt>=0);

== matlab function RealSongControl/DSPBlock/BoutCounter/CorrectDelayedPulseGenerator forRecordingEnableSignal/Delayed TTL generator ==
  data: trig input double; out output double; delays input double; width input double
function out = fcn(trig,delays,width)
% return delayed broader TTL pulse, 
% 
% 
persistent cnt_for_delay; % counter for delays
persistent width_cnt;


if isempty(cnt_for_delay)
    cnt_for_delay=-inf(size(trig));
    width_cnt=zeros(size(trig));
end

cnt_for_delay=cnt_for_delay-1;
trigind=(trig>0);

width_cnt(cnt_for_delay==0)=width; % set width counter.
cnt_for_delay(trigind)=delays(trigind)+1; % plus one, so that delays=0 can trigger next time.

width_cnt=width_cnt-1;    
out=(width_cnt>0);

== matlab function RealSongControl/DSPBlock/FeatureBasedTrigger/ResettableSyllableCounter/MATLAB Function ==
  data: x input double; y output double; reset input double
function y = resettable_counter(x,reset)
%#codegen

persistent tmp;

if isempty(tmp)
    tmp=uint8(0);
end

tmp=tmp+x;

if (reset)
    tmp=uint8(0);
end

y = tmp;

== matlab function RealSongControl/triggered_dynamic_Pulse/Triggered_dynamic_pulse ==
  data: trig input double; out output double; delay input double; pulse_dur input double; inter_pulse_interval input double; burst_dur input double; ref input double
function out = trig_dynamic_pulse(trig,delay,pulse_dur,inter_pulse_interval,burst_dur,ref)
%#eml
% once triggered, start generating dynamic pulse with
%       pulse_dur
%        <->
%        ___        ___        ___
% ______|   |______|   |______|   |______
% delay <--------->  
%         inter_pulse_interval
%       <----------burst duration-------->
%  out = 1 if (cnt>delay) AND (mod(cnt-delay,inter_pulse_interval)<pulse_dur)
%             AND (cnt-delay<burst_dur)
%  else out=0;
% It does not triggered again unless delay + ref counts has passed from thr
% trigger.
% by KH 20120426


persistent cnt; % counter 
persistent ref_cnt; % refractoriness counter 


if isempty(cnt)
    cnt=2*ref;
    ref_cnt=2*ref;
end

if (trig>0) && (ref_cnt>ref)
    cnt=0;
    ref_cnt=0;
end



scnt=cnt-delay; % shifted cnt

out = (scnt>=0)&&(mod(scnt,inter_pulse_interval)<pulse_dur)&&(scnt<burst_dur)&&(scnt<ref);
%  out = 1 if (cnt>delay) AND (mod(cnt-delay,inter_pulse_interval)<=pulse_dur)
%             AND (cnt-delay<burst_dur)

cnt=cnt+1;
ref_cnt=ref_cnt+1;

if scnt>=2*ref
    cnt=2*ref+delay;
    ref_cnt=2*ref+delay;
end

== matlab function RealSongControl/Triggered_1ms_TTL/Triggered_dynamic_pulse ==
  data: trig input double; out output double; delay input double; pulse_dur input double; inter_pulse_interval input double; burst_dur input double; ref input double
function out = trig_dynamic_pulse(trig,delay,pulse_dur,inter_pulse_interval,burst_dur,ref)
%#eml
% once triggered, start generating dynamic pulse with
%       pulse_dur
%        <->
%        ___        ___        ___
% ______|   |______|   |______|   |______
% delay <--------->  
%         inter_pulse_interval
%       <----------burst duration-------->
%  out = 1 if (cnt>delay) AND (mod(cnt-delay,inter_pulse_interval)<pulse_dur)
%             AND (cnt-delay<burst_dur)
%  else out=0;
% It does not triggered again unless delay + ref counts has passed from thr
% trigger.
% by KH 20120426


persistent cnt; % counter 
persistent ref_cnt; % refractoriness counter 


if isempty(cnt)
    cnt=2*ref;
    ref_cnt=2*ref;
end

if (trig>0) && (ref_cnt>ref)
    cnt=0;
    ref_cnt=0;
end



scnt=cnt-delay; % shifted cnt

out = (scnt>=0)&&(mod(scnt,inter_pulse_interval)<pulse_dur)&&(scnt<burst_dur)&&((delay+ref_cnt)<ref);
%  out = 1 if (cnt>delay) AND (mod(cnt-delay,inter_pulse_interval)<=pulse_dur)
%             AND (cnt-delay<burst_dur)

cnt=cnt+1;
ref_cnt=ref_cnt+1;

if ref_cnt>=2*ref
    cnt=2*ref;
    ref_cnt=2*ref;
end

== matlab function OscilloAntidromic/CorrectPulseGenerator/Delayed TTL generator ==
  data: trig input double; out output double; delays input double; width input double
function out = fcn(trig,delays,width)
% return delayed broader TTL pulse, 
% 
% 
persistent cnt_for_delay; % counter for delays
persistent width_cnt;


if isempty(cnt_for_delay)
    cnt_for_delay=-inf(size(trig));
    width_cnt=zeros(size(trig));
end

cnt_for_delay=cnt_for_delay-1;
trigind=(trig>0);

width_cnt(cnt_for_delay==0)=width; % set width counter.
cnt_for_delay(trigind)=delays(trigind)+1; % plus one, so that delays=0 can trigger next time.

width_cnt=width_cnt-1;    
out=(width_cnt>0);

== matlab function OscilloAntidromic/triggered_dynamic_Pulse/Triggered_dynamic_pulse ==
  data: trig input double; out output double; delay input double; pulse_dur input double; inter_pulse_interval input double; burst_dur input double; ref input double
function out = trig_dynamic_pulse(trig,delay,pulse_dur,inter_pulse_interval,burst_dur,ref)
%#eml
% once triggered, start generating dynamic pulse with
%       pulse_dur
%        <->
%        ___        ___        ___
% ______|   |______|   |______|   |______
% delay <--------->  
%         inter_pulse_interval
%       <----------burst duration-------->
%  out = 1 if (cnt>delay) AND (mod(cnt-delay,inter_pulse_interval)<pulse_dur)
%             AND (cnt-delay<burst_dur)
%  else out=0;
% It does not triggered again unless delay + ref counts has passed from thr
% trigger.
% by KH 20120426


persistent cnt; % counter 
persistent ref_cnt; % refractoriness counter 


if isempty(cnt)
    cnt=2*ref;
    ref_cnt=2*ref;
end

% If triggered and only if refractoriness is over, we can re-trigger.
if (trig>0) && (ref_cnt>ref)
    cnt=0;
    ref_cnt=0;
end



scnt=cnt-delay; % shifted cnt

out = (scnt>=0)&&(mod(scnt,inter_pulse_interval)<pulse_dur)&&(scnt<burst_dur)&&((delay+ref_cnt)<ref);
%  out = 1 if (cnt>delay) AND (mod(cnt-delay,inter_pulse_interval)<=pulse_dur)
%             AND (cnt-delay<burst_dur)

cnt=cnt+1;
ref_cnt=ref_cnt+1;

if ref_cnt>=2*ref
    cnt=2*ref;
    ref_cnt=2*ref;
end

== matlab function OscilloAntidromic/triggered_pulse_family/Triggered_pulse_family ==
  data: trig input double; lowamp input double; interval input double; highamp input double; out output double; delay input double; pulse_dur input double; inter_pulse_interval input double; burst_dur input double; ref input double; absout output double
function [out,absout] = trig_pulse_family(trig,lowamp,interval,highamp,delay,pulse_dur,inter_pulse_interval,burst_dur,ref)
%#eml
% once triggered, start generating dynamic pulse with
%       pulse_dur
%        <->        ___  amp(2)
%  amp(1)___       |   |       
% ______|   |______|   |______    ______
%       <--------->           |   |
%      inter_pulse_interval   |___| amp(3)...
% delay
% <---->        
%       <----------burst duration-------->
% 
% 
% 
%  out = amp if (cnt>delay) AND (mod(cnt-delay,inter_pulse_interval)<pulse_dur)
%             AND (cnt-delay<burst_dur);
%  absout is 1 when generating output.
%  else out=0;
% 
% amp is 1x ceil(burst_duration/inter_pulse_interval) vector.
% otherwise, when there is no corresponding amp value for a pulse, it just
% use the amp(end) value.
% 
% 
% It does not triggered again unless delay + ref counts has passed from the
% trigger.
% by KH 20120426


persistent cnt; % counter 
persistent ref_cnt; % refractoriness counter 


if isempty(cnt)
    cnt=2*ref;
    ref_cnt=2*ref;
end

% If triggered and only if refractoriness is over, we can re-trigger.
if (trig>0) && (ref_cnt>ref)
    cnt=0;
    ref_cnt=0;
end



scnt=cnt-delay; % shifted cnt

do_pulse =   (scnt>=0)&&... % delay period is over, 
        (mod(scnt,inter_pulse_interval)<pulse_dur)&&... % and shifted-count is within pulse-dur,
        (scnt<burst_dur);   % and shifted-count must be within the total burst duration, 
%         ((delay+ref_cnt)<ref);  % and I think we do not need this condition...


amp_index=ceil(scnt/inter_pulse_interval);
amp=lowamp+(amp_index-1)*interval; 

if (do_pulse)
    if amp>highamp
        out=highamp/1000; % 10H nA/V and H=0.1; 1nA/V. 
    else
        out=amp/1000;     % 10H nA/V and H=0.1; 1nA/V. 
    end
    absout=1.0;
else
    absout=1.0;
    out=0.0;
end
    
    
cnt=cnt+1;
ref_cnt=ref_cnt+1;

if ref_cnt>=2*ref
    cnt=2*ref;
    ref_cnt=2*ref;
end

== matlab function RealSongControl/DSPBlock/FeatureBasedTrigger/RndCatchMainGateWindow/CorrectDelayedPulseGenerator1/Delayed TTL generator ==
  data: trig input double; out output double; delays input double; width input double
function out = fcn(trig,delays,width)
% return delayed broader TTL pulse.
% Trigger always reset the delay counter, therefore, 
% when two trigger occurs, first one can be just forgotten. 
% by KH.

persistent cnt_for_delay; % counter for delays
persistent width_cnt;


if isempty(cnt_for_delay)
    cnt_for_delay=-inf(size(trig));
    width_cnt=zeros(size(trig));
end

cnt_for_delay=cnt_for_delay-1;
trigind=(trig>0);

width_cnt(cnt_for_delay==0)=width; % set width counter.
cnt_for_delay(trigind)=delays(trigind)+1; % plus one, so that delays=0 can trigger next time.

width_cnt=width_cnt-1;    
out=(width_cnt>0);

== matlab function RealSongControl/DSPBlock/YIN_FF_estim/YIN_FF ==
  data: x input double; F0 output double; Fs input double; W_index input double; lag_index input double
function F0 = YIN_FF_estimater(x,Fs,W_index,lag_index)
%#codegen
% Copy of function [FF,t]=YIN_FF_estimator(x,Fs,varargin)
% Estimate fundamental frequency based on YIN-YANG algorithm
% proposed in Alain de Cheveigne and Hideki Kawahara,
% J. Acouts. Soc. Am, 111 (4), pp. 1917-1930, 2002.
%
% Implemented in MATLAB by Kosuke Hamaguchi, 2013.4.4.
% Note: the last step6, search for best local estimate was not implemented.
% 
%
% Usage1)
% [FF,t]=YIN_FF_estimator(x,Fs);
% Input)
% x     : input singal (a vector).
% Fs    : sampling rate.
%
% Output)
% FF    : YIN estimate of fundamental frequency, estimated at every 1ms,
%       using default window size 2.5ms (suitable for zebra finch), and
%       search window lagT = 5ms.
% t     : time points.
%
% Usage2)
% [FF,t]=YIN_FF_estimator(x,Fs,winT,lagT,t);
%
% winT  : window size in ms. Default is 2.5ms (looking for FF > 400Hz).
% lagT  : length of search. Needs to be twice longer than the longest
%         expected period. Default is 5ms.
% t     : vector of time points to estimate FF.
%         t is placed at the center of winT, thus actual window is [t-winT/2,t+winT/2];
%         The sound in the window is compared to future time windows
%         until [t-winT/2+lagT t+winT/2+lagT].
%
%         If you prefer to compare the time in the past,
%         like actual real-time FF detection case,
%         use option 'backward' as below;
%
%
% Usage3)
% [FF,t]=YIN_FF_estimator(x,Fs,winT,lagT,t,threshold,option);
%
% threshold: absolute threshold to find minimum of "cumulative-mean
% normalized difference function". Default is 0.1.
%
% option: direction of search.
%       : 'forward' compares the time in the future (Default).
%       : 'backward' compares the time in the past
%          (real-time FF detection use this).
%
%
%% example)
% % [x,Fs]=wavread('C:\home\Experiments\RealSong_ChronicData\grn1028m\SongData\grn1028m_41367.64484782_4_3_17_54_44.wav');
%
% [x,Fs]=wavread('C:\home\Experiments\AivAxonStim_VTA_withErin\org1008m\org1008m_2013_03_11_115010.wav');
%
% [B,A]=ellip(4,.1,50,[600,10000]/(Fs/2));
% x=filtfilt(B,A,x);
%
% t=linspace(0,length(x)/Fs,length(x));
% figure(1);clf;
%  [y,f,t,p] = spectrogram(x,256,250,1024,Fs);
%  imagesc(t,f,10*log10(abs(p)));set(gca,'YDir','normal');
%
%
% winT=4; % ms % lowest resolution is 1000/winT [Hz].
% lagT=2; % ms % needs to be twice longer than expected longest period.
% threshold= 0.1; % threshold for cumulative mean normalized difference function.
% option = 'forward';
%
% t=[]; % use default, 1ms intervals.
% [FF,t]=YIN_FF_estimator(x,Fs,winT,lagT,t,threshold,option);
%
% ca=caxis; caxis([+100 -5]+ca);
% hold on; plot(t,FF,'g');
%%
% 
% 
% in simulink version, following parameters are pre-computed.
% nx = length(x);
% nW=ceil(winT/1000*Fs);
% nlag=ceil(lagT/1000*Fs);
% 
% W_index=0:(nW-1);
% W_index = nx-W_index;
% 
% lag_index = nW+[0:(nlag-1)];
% lag_index = nx-lag_index;


xw=x(W_index);
xl=x(lag_index);
nlag=length(lag_index);

% hankel matrix to generate time-lag matrix.
d= hankel(xw,xl);
d=d-repmat(xw(:),1,nlag);

d=sum(d.^2,1);
aved =cumsum(d)./[1:nlag];
cumd = d./aved;
cumd(1)=1;

threshold=0.1;

% More bias on first dip below absolute threshold.
cumd_less_thresh=find(cumd<threshold,3,'first');
if isempty(cumd_less_thresh) % No minimum lower than threshold, then take global minimum.
    [cumd_min,cumd_min_ind]=min(cumd);
else % If there is a minimum lower than threshold,
    
    [cumd_min,cumd_min_ind]=min(cumd(cumd_less_thresh));
    cumd_min_ind=cumd_less_thresh(cumd_min_ind);
end

% toc

df=1;
% Calculate parabolic estimate (pe);
if (cumd_min_ind==1)|| (cumd_min_ind==length(cumd))
    pe = 1;
    F0=0;
else
    dy1 = cumd(cumd_min_ind-1)-cumd(cumd_min_ind);
    dy2 = cumd(cumd_min_ind)-cumd(cumd_min_ind+1);
    
    a = -(dy1-dy2)/(2*df^2);
    b = dy1/df - 2 * a * (cumd_min_ind-0.5);
    pe = -b/(2*a);
    c = cumd(cumd_min_ind-1)+a*(cumd_min_ind-1)^2+b*(cumd_min_ind-1);
    
    F0=Fs/(pe-1);   
end
